simulink model "pathPlanningTest"  (R2022a)
settings: Solver=VariableStepAuto  StartTime=0.0  StopTime=1000  RelTol=1e-3
model workspace (MAT data in the model file):
  Sig = Simulink.Signal
  Sig.DataType = 'auto'
  Sig.Dimensions = -1
  Sig.DimensionsMode = 'auto'
  Sig.Complexity = 'auto'
  Sig.SampleTime = -1
  Sig.SamplingMode = 'auto'
  fg = 0.14
values from neighbouring files (symbols this model uses):
  dphi = [0]    [Trajectory_Generate.m]    (also in Trajectory_Generate_Circumference.m = zeros([1 length(t)]); Trajectory_Generate_Line.m = zeros([1 length(t)]); Trajectory_Generate_Straigth.m = zeros([1 length(t)]); teste.m = [])
  iteractions = length(x)    [Trajectory_Generate.m]    (also in Trajectory_Generate_Circumference.m = length(phi)-1; Trajectory_Generate_Line.m = length(phi); Trajectory_Generate_Straigth.m = length(dphi)-1; teste.m = length(phi))
  v = [0]    [Trajectory_Generate.m]    (also in Trajectory_Generate_Circumference.m = zeros([1 length(t)]); Trajectory_Generate_Line.m = zeros([1 length(t)]); Trajectory_Generate_Straigth.m = zeros([1 length(t)]); cubicTrajectory.m = zeros(1,length(t)))
libraries: robotmobilelib x1
settings Model: Creator=The MathWorks, Inc.  LastModifiedBy=Gabriel-PC
settings SolverCC: AlgebraicLoopSolver=TrustRegion
settings DebuggingCC: UnconnectedInputMsg=warning  UnconnectedOutputMsg=warning  UnconnectedLineMsg=warning  SymbolicDimsDataTypeCodeGenerationDiagnostic=none  SFMachineParentedDataDiag=warning
settings RTWCC: DLArmComputeVersion=19.05

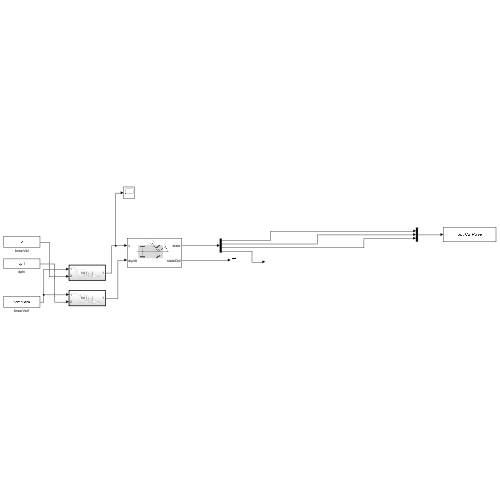
[thumbnail: Simulink's stored preview of the top-level diagram]
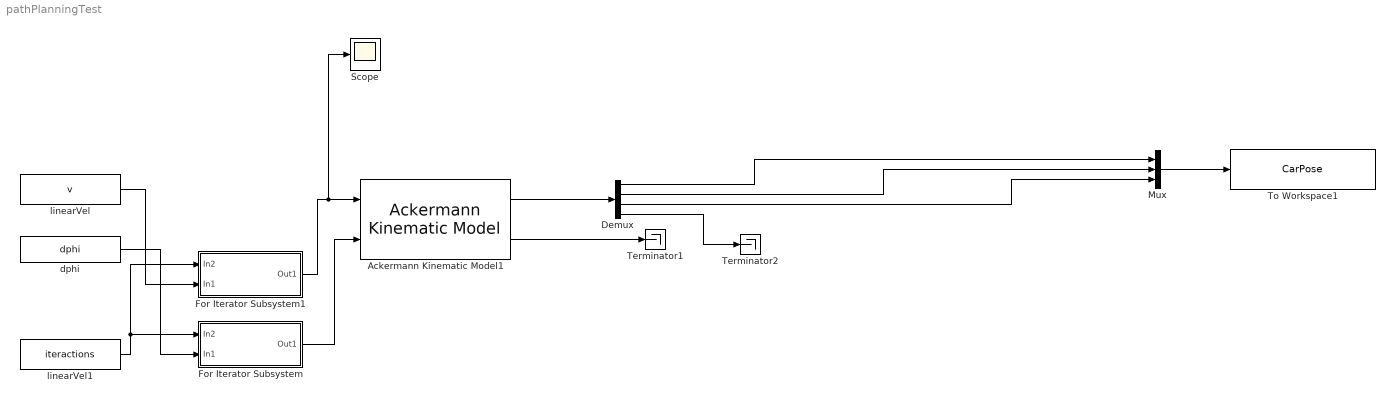
== system pathPlanningTest ==
  Ackermann Kinematic Model1 : robotmobilelib/Ackermann Kinematic Model  WheelBase=wheelbase  VehicleSpeedRange=[-inf inf]  MaxSteeringAngle=pi/4  InitialState=initState  SimulateUsing=Interpreted execution
      settings: SourceProductBaseCode=RO
  Demux : Demux
  For Iterator Subsystem : Subsystem  TreatAsAtomicUnit=on
  For Iterator Subsystem1 : Subsystem  TreatAsAtomicUnit=on
  Mux : Mux  Inputs=3
  Scope : Scope
  Terminator1 : Terminator
  Terminator2 : Terminator
  To Workspace1 : ToWorkspace  VariableName=CarPose  SampleTime=-1
  dphi : Constant  Value=dphi
  linearVel : Constant  Value=v
  linearVel1 : Constant  Value=iteractions
  wires:
  Demux/1 -> Mux/1
  Demux/2 -> Mux/2
  Demux/3 -> Mux/3
  Mux/1 -> To Workspace1/1
  dphi/1 -> For Iterator Subsystem/2(In1)
  linearVel/1 -> For Iterator Subsystem1/2(In1)
  linearVel1/1 -> For Iterator Subsystem/1(In2), For Iterator Subsystem1/1(In2)
  Ackermann Kinematic Model1/1 -> Demux/1
  Ackermann Kinematic Model1/2 -> Terminator1/1
  For Iterator Subsystem1/1(Out1) -> Scope/1, Ackermann Kinematic Model1/1
  For Iterator Subsystem/1(Out1) -> Ackermann Kinematic Model1/2
  Demux/4 -> Terminator2/1

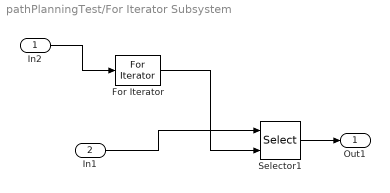
== system pathPlanningTest/For Iterator Subsystem ==
  In2 : Inport
  In1 : Inport  Port=2
  For Iterator : ForIterator  IterationSource=external  IndexMode=Zero-based
  Selector1 : Selector  NumberOfDimensions=2  IndexMode=Zero-based  InputPortWidth=3  IndexOptions=Select all,Index vector (port)  Indices=[1 3],1  OutputSizes=1,1
  Out1 : Outport
  wires:
  In2/1 -> For Iterator/1
  For Iterator/1 -> Selector1/2
  In1/1 -> Selector1/1
  Selector1/1 -> Out1/1

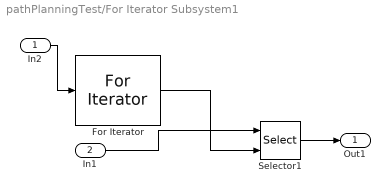
== system pathPlanningTest/For Iterator Subsystem1 ==
  In2 : Inport
  In1 : Inport  Port=2
  For Iterator : ForIterator  IterationSource=external  IndexMode=Zero-based
  Selector1 : Selector  NumberOfDimensions=2  IndexMode=Zero-based  InputPortWidth=3  IndexOptions=Select all,Index vector (port)  Indices=[1 3],1  OutputSizes=1,1
  Out1 : Outport
  wires:
  In2/1 -> For Iterator/1
  In1/1 -> Selector1/1
  Selector1/1 -> Out1/1
  For Iterator/1 -> Selector1/2
